simulink model "TorqueControlConfig"  (R2023b)
settings: Solver=VariableStepAuto  StartTime=0.0  StopTime=20  RelTol=1e-3
PostLoadFcn:
  | run('ParametricRobotLoader.m')
  | run('ParametricRobotParameters');
  | TsCtrl=0.005
  | Config.Mode=ones(1,6)
  | Config.Value = zeros(1,6)
undefined symbols (not defined in the file): ctrlLowerLimit, ctrlUpperLimit
libraries: nesl_utility x19, fl_lib x6, slpidlib x6, sm_lib x3, simulink x2, robotmaniplib x1
(part 2 of 2)

== system TorqueControlConfig/Robot Subsystem/Sensor Data/Subsystem15 ==
  " " : Inport
  Demux1 : Demux  Outputs=3
  "  " : Outport
  wires:
  Demux1/3 -> "  "/1
  " "/1 -> Demux1/1

== system TorqueControlConfig/Robot Subsystem/Sensor Data/Subsystem16 ==
  " " : Inport
  Demux1 : Demux  Outputs=3
  "  " : Outport
  wires:
  " "/1 -> Demux1/1
  Demux1/3 -> "  "/1

== system TorqueControlConfig/Robot Subsystem/Sensor Data/Subsystem17 ==
  " " : Inport
  Demux1 : Demux  Outputs=3
  "  " : Outport
  wires:
  Demux1/3 -> "  "/1
  " "/1 -> Demux1/1

== system TorqueControlConfig/Robot Subsystem/Sensor Data/Subsystem2 ==
  " " : Inport
  Demux1 : Demux  Outputs=3
  "  " : Outport
  wires:
  " "/1 -> Demux1/1
  Demux1/1 -> "  "/1

== system TorqueControlConfig/Robot Subsystem/Sensor Data/Subsystem3 ==
  " " : Inport
  Demux1 : Demux  Outputs=3
  "  " : Outport
  wires:
  Demux1/1 -> "  "/1
  " "/1 -> Demux1/1

== system TorqueControlConfig/Robot Subsystem/Sensor Data/Subsystem4 ==
  " " : Inport
  Demux1 : Demux  Outputs=3
  "  " : Outport
  wires:
  " "/1 -> Demux1/1
  Demux1/1 -> "  "/1

== system TorqueControlConfig/Robot Subsystem/Sensor Data/Subsystem5 ==
  " " : Inport
  Demux1 : Demux  Outputs=3
  "  " : Outport
  wires:
  Demux1/1 -> "  "/1
  " "/1 -> Demux1/1

== system TorqueControlConfig/Robot Subsystem/Sensor Data/Subsystem6 ==
  " " : Inport
  Demux1 : Demux  Outputs=3
  "  " : Outport
  wires:
  " "/1 -> Demux1/1
  Demux1/2 -> "  "/1

== system TorqueControlConfig/Robot Subsystem/Sensor Data/Subsystem7 ==
  " " : Inport
  Demux1 : Demux  Outputs=3
  "  " : Outport
  wires:
  Demux1/2 -> "  "/1
  " "/1 -> Demux1/1

== system TorqueControlConfig/Robot Subsystem/Sensor Data/Subsystem8 ==
  " " : Inport
  Demux1 : Demux  Outputs=3
  "  " : Outport
  wires:
  " "/1 -> Demux1/1
  Demux1/2 -> "  "/1

== system TorqueControlConfig/Robot Subsystem/Sensor Data/Subsystem9 ==
  " " : Inport
  Demux1 : Demux  Outputs=3
  "  " : Outport
  wires:
  Demux1/2 -> "  "/1
  " "/1 -> Demux1/1
